simulink model "Sample"  (R2020a)
settings: Solver=FixedStepAuto  StartTime=0.0  StopTime=Inf  RelTol=1e-3
settings Model: Creator=eisuk  LastModifiedBy=eisuk
settings SolverCC: PositivePriorityOrder=on
settings DataIOCC: ReturnWorkspaceOutputs=off
settings OptimizationCC: EnhancedBackFolding=on  PassReuseOutputArgsAs=Individual arguments  ZeroExternalMemoryAtStartup=off  ZeroInternalMemoryAtStartup=off  MaxStackSize=64  OptimizeBlockOrder=speed  DifferentSizesBufferReuse=on  OptimizationCustomize=off  EfficientTunableParamExpr=on
settings DebuggingCC: ParameterTunabilityLossMsg=error
settings HardwareCC: ProdBitPerPointer=32  ProdBitPerSizeT=32  ProdBitPerPtrDiffT=32  ProdLargestAtomicInteger=Long  ProdLargestAtomicFloat=Double  ProdWordSize=32  ProdLongLongMode=on  ProdHWDeviceType=ARM Compatible->ARM Cortex
settings RTWCC: SystemTargetFile=ert.tlc  HardwareBoard=Raspberry Pi  TemplateMakefile=ert_default_tmf  Toolchain=GNU GCC Raspberry Pi  BuildConfiguration=Faster Runs
settings CodeAppCC: ForceParamTrailComments=on  IgnoreCustomStorageClasses=off  OperatorAnnotations=on  SimulinkDataObjDesc=on  SFDataObjDesc=on  InsertBlockDesc=on
settings ERTTargetCC: SupportVariableSizeSignals=on

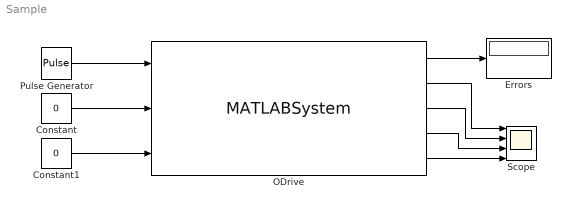
== system Sample ==
  Constant : Constant  Value=0
  Constant1 : Constant  Value=0
  Errors : Display
      settings: Format=hex (Stored Integer)
  ODrive : MATLABSystem  System=ODriveRasPi  SampleTime=0.01  isPort=off  portName=/dev/ttyACM0  serial=123456789ABC  isAxis0=on  ctrlMode0=Position  isInCpr0=off  isVelRamp0=off  watchdog0=0  isExternal0=off  posGain0=20.0  velGain0=0.0005  velIGain0=0.001  velLimit0=20000.0  velLimitTol0=1.2  velRampRate0=10000.0  isAxis1=off  ctrlMode1=Position  isInCpr1=off  isVelRamp1=off  watchdog1=0  isExternal1=off  posGain1=20.0  velGain1=0.0005  velIGain1=0.001  velLimit1=20000.0  velLimitTol1=1.2  velRampRate1=10000.0
      mask Type: ODriveRasPi
      mask Display:
      | disp(['ODrive' char(10) '' char(10) 'Serial: 123456789ABC' char(10) '' char(10) 'M0: Position control' char(10) 'M1: Disable']);
      | port_label('input',1,'M0 position ref');
      | port_label('input',2,'M0 velocity ref');
      | port_label('input',3,'M0 current ref');
      | port_label('output',1,'Axis error');
      | port_label('output',2,'M0 position act');
      | port_label('output',3,'M0 velocity act');
      | port_label('output',4,'M0 current act');
      | port_label('output',5,'M0 vel integral act');
  Pulse Generator : DiscretePulseGenerator  Amplitude=100000  Period=100  PulseWidth=50  PhaseDelay=1  SampleTime=0.1
  Scope : Scope  NumInputPorts=4
  wires:
  ODrive/1 -> Errors/1
  ODrive/2 -> Scope/1
  ODrive/3 -> Scope/2
  ODrive/5 -> Scope/4
  ODrive/4 -> Scope/3
  Constant/1 -> ODrive/2
  Constant1/1 -> ODrive/3
  Pulse Generator/1 -> ODrive/1
